simulink model "SFunctionTest1"  (R2023a)
settings: Solver=VariableStepAuto  StartTime=0.0  StopTime=10.0  RelTol=1e-3
libraries: simulink x1
settings Model: Creator=涂钱龙  LastModifiedBy=涂钱龙
settings OptimizationCC: DefaultParameterBehavior=Inlined  EnhancedBackFolding=on  PassReuseOutputArgsAs=Individual arguments  ZeroExternalMemoryAtStartup=off  ZeroInternalMemoryAtStartup=off  OptimizeBlockOrder=speed  DifferentSizesBufferReuse=on  OptimizationCustomize=off  EfficientTunableParamExpr=on
settings DebuggingCC: ParameterTunabilityLossMsg=error
settings HardwareCC: TargetBitPerPointer=64  TargetBitPerSizeT=64  TargetBitPerPtrDiffT=64  TargetLongLongMode=on  TargetIntDivRoundTo=Zero  TargetEndianess=LittleEndian  TargetWordSize=64  TargetHWDeviceType=MATLAB Host
settings SFSimCC: MATLABDynamicMemAlloc=off
settings RTWCC: Description=Embedded Coder  SystemTargetFile=ert.tlc  GenCodeOnly=on  TemplateMakefile=ert_default_tmf  RTWVerbose=off
settings CodeAppCC: ForceParamTrailComments=on  IgnoreCustomStorageClasses=off  OperatorAnnotations=on  SimulinkDataObjDesc=on  SFDataObjDesc=on  InsertBlockDesc=on
settings ERTTargetCC: GenerateSampleERTMain=on  InlinedParameterPlacement=NonHierarchical  ERTCustomFileTemplate=example_file_process.tlc

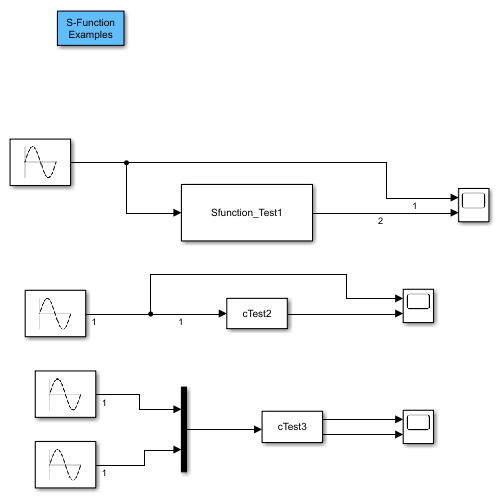
[thumbnail: Simulink's stored preview of the top-level diagram]
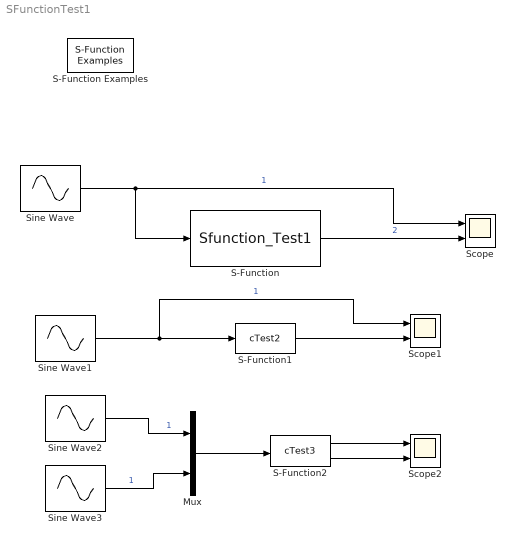
== system SFunctionTest1 ==
  Mux : Mux  Inputs=2
  S-Function : S-Function  FunctionName=Sfunction_Test1  Parameters=5  SFunctionDeploymentMode=off  EnableBusSupport=off
  S-Function Examples : simulink/User-Defined Functions/S-Function Examples
  S-Function1 : S-Function  FunctionName=cTest2  Parameters=2  SFunctionDeploymentMode=off  EnableBusSupport=off
  S-Function2 : S-Function  FunctionName=cTest3  Parameters=2,3,4  SFunctionDeploymentMode=off  EnableBusSupport=off
  Scope : Scope  NumInputPorts=2
  Scope1 : Scope  NumInputPorts=2
  Scope2 : Scope  NumInputPorts=2
  Sine Wave : Sin  SampleTime=0
  Sine Wave1 : Sin  SampleTime=0
  Sine Wave2 : Sin  SampleTime=0
  Sine Wave3 : Sin  Phase=pi  SampleTime=0
  wires:
  Sine Wave/1 -> Scope/1, S-Function/1  "1"
  S-Function/1 -> Scope/2  "2"
  Sine Wave1/1 -> S-Function1/1, Scope1/1  "1"
  S-Function1/1 -> Scope1/2
  Sine Wave2/1 -> Mux/1  "1"
  Sine Wave3/1 -> Mux/2  "1"
  Mux/1 -> S-Function2/1
  S-Function2/1 -> Scope2/1
  S-Function2/2 -> Scope2/2
